simulink model "test_zumo_orientation_ketan"  (R2014b)
settings: Solver=ode3  StartTime=0.0  StopTime=10.0  RelTol=1e-3
InitFcn:
  | prepareCurrentFolderForZumo;
  | load MagnetometerBus;
libraries: arduinolib x2, etargetslib x2, ZumoBotLib x1
settings Model: ExtModeTrigDuration=2  Creator=sandip  LastModifiedBy=sandip
settings OptimizationCC: OptimizeModelRefInitCode=on  LifeSpan=1
settings DebuggingCC: UnderspecifiedInitializationDetection=Classic  MergeDetectMultiDrivingBlocksExec=none  SolverPrmCheckMsg=none
settings HardwareCC: ProdBitPerInt=16  ProdBitPerPointer=8  ProdIntDivRoundTo=Zero  ProdEndianess=LittleEndian  ProdWordSize=8  ProdHWDeviceType=Atmel->AVR
settings RTWCC: SystemTargetFile=realtime.tlc  GenerateMakefile=off  TemplateMakefile=realtime.tmf  Description=Run on Target Hardware  RTWVerbose=off  ProcessScript=realtime_make_rtw_hook
settings STFCustomTargetCC: TargetLibSuffix=.a  GenerateSampleERTMain=on  ERTCustomFileBanners=on  SupportNonInlinedSFcns=off  SupportVariableSizeSignals=on  MATLABClassNameForMDSCustomization=Simulink.SoftwareTarget.ERTCustomization  GRTInterface=off  SystemTargetFile=realtime.tlc
settings ERTTargetCC: GenerateSampleERTMain=on  ParMdlRefBuildCompliant=off  CompOptLevelCompliant=off  ConcurrentExecutionCompliant=off  CombineOutputUpdateFcns=off  ERTFirstTimeCompliant=off  SupportContinuousTime=on  SupportVariableSizeSignals=on  ModelStepFunctionPrototypeControlCompliant=off  CPPClassGenCompliant=off  ExtModeTransport=3  ExtModeMexFile=ext_serial_win32_comm  ExtModeMexArgs=0 1 9600  InlinedParameterPlacement=NonHierarchical  ERTSrcFileBannerTemplate=realtime_code_template.cgt  ERTHdrFileBannerTemplate=realtime_code_template.cgt  ERTDataSrcFileTemplate=realtime_code_template.cgt  ERTDataHdrFileTemplate=realtime_code_template.cgt  ERTCustomFileTemplate=realtime_file_process.tlc

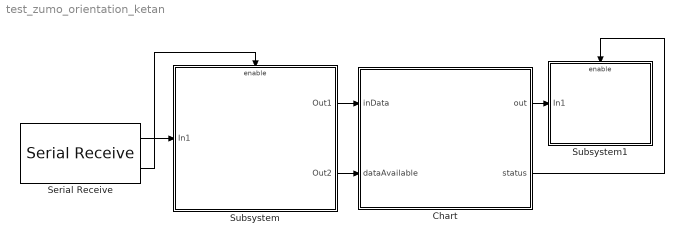
== system test_zumo_orientation_ketan ==
  Chart : Stateflow chart  TreatAsAtomicUnit=on
  Serial Receive : arduinolib/Serial Receive  portNumber=0  showOutStatus=on  sampleTime=0.01  blockPlatform=arduino
  Subsystem : Subsystem
  Subsystem1 : Subsystem
  wires:
  Serial Receive/2 -> Subsystem/Enable
  Subsystem/1(Out1) -> Chart/1(inData)
  Subsystem/2(Out2) -> Chart/2(dataAvailable)
  Chart/1(out) -> Subsystem1/1(In1)
  Chart/2(status) -> Subsystem1/Enable
  Serial Receive/1 -> Subsystem/1(In1)

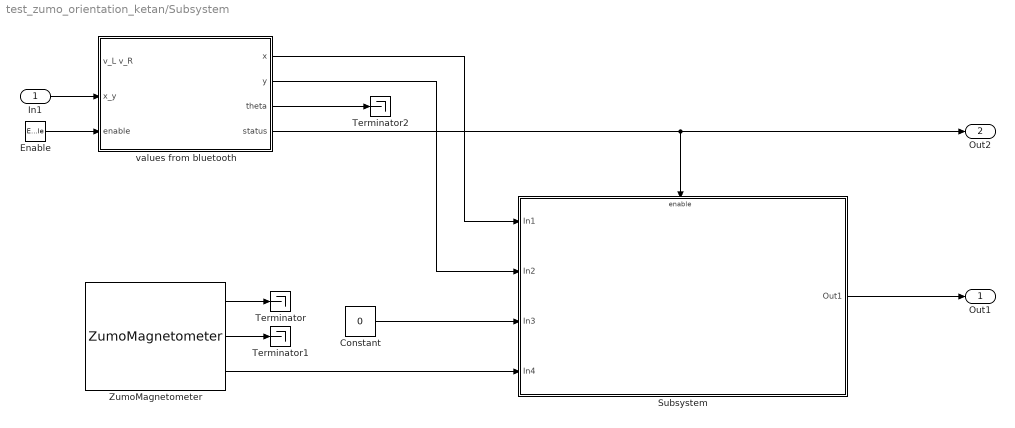
== system test_zumo_orientation_ketan/Subsystem ==
  In1 : Inport
  Enable : EnablePort  ShowOutputPort=on
  Constant : Constant  Value=0
  Subsystem : Subsystem
  Terminator : Terminator
  Terminator1 : Terminator
  Terminator2 : Terminator
  ZumoMagnetometer : ZumoBotLib/ZumoMagnetometer  sampletime_lsm=0.01  debug_lsm=off  minX_lsm=-2048  maxX_lsm=2048  minY_lsm=-2048  maxY_lsm=2048  minZ_lsm=-4096  maxZ_lsm=4096
      link override S-Function Builder: Parameters=sampletime_lsm,boolean(debug_lsm),minX_lsm,maxX_lsm,minY_lsm,maxY_lsm,minZ_lsm,boolean(maxZ_lsm)
  "values from bluetooth " : Subsystem  VariantControl=bluetoothComm==1
  Out1 : Outport
  Out2 : Outport  Port=2  OutputWhenDisabled=reset  InitialOutput=0
  wires:
  ZumoMagnetometer/2 -> Terminator1/1
  ZumoMagnetometer/1 -> Terminator/1
  "values from bluetooth "/3(theta) -> Terminator2/1
  In1/1 -> "values from bluetooth "/2(x_y)
  "values from bluetooth "/1(x) -> Subsystem/1(In1)
  "values from bluetooth "/2(y) -> Subsystem/2(In2)
  Constant/1 -> Subsystem/3(In3)
  ZumoMagnetometer/3 -> Subsystem/4(In4)
  "values from bluetooth "/4(status) -> Subsystem/Enable, Out2/1
  Subsystem/1(Out1) -> Out1/1
  Enable/1 -> "values from bluetooth "/3(enable)

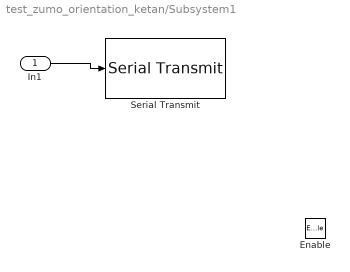
== system test_zumo_orientation_ketan/Subsystem1 ==
  In1 : Inport
  Enable : EnablePort
  Serial Transmit : arduinolib/Serial Transmit  portNumber=0  blockPlatform=arduino
  wires:
  In1/1 -> Serial Transmit/1

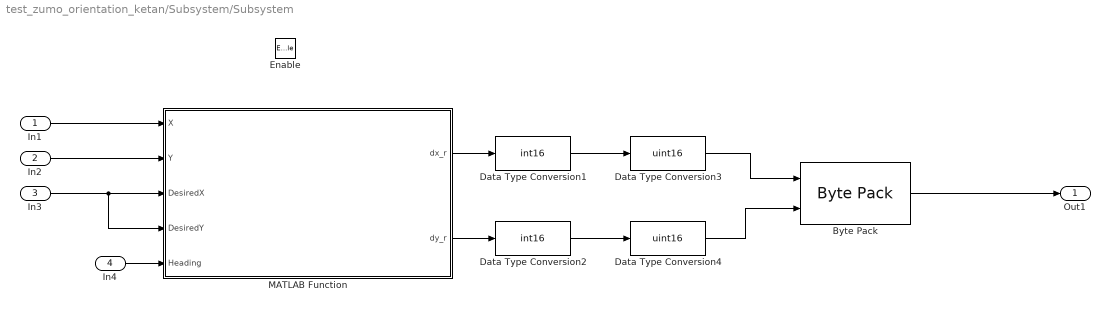
== system test_zumo_orientation_ketan/Subsystem/Subsystem ==
  In1 : Inport
  In2 : Inport  Port=2
  In3 : Inport  Port=3
  In4 : Inport  Port=4
  Enable : EnablePort
  Byte Pack : etargetslib/Byte Pack  datatypes={'uint16','uint16'}  byteAlign=1
  Data Type Conversion1 : DataTypeConversion  OutDataTypeStr=int16
  Data Type Conversion2 : DataTypeConversion  OutDataTypeStr=int16
  Data Type Conversion3 : DataTypeConversion  OutDataTypeStr=uint16  ConvertRealWorld=Stored Integer (SI)
  Data Type Conversion4 : DataTypeConversion  OutDataTypeStr=uint16  ConvertRealWorld=Stored Integer (SI)
  MATLAB Function : MATLAB Function  TreatAsAtomicUnit=on
  Out1 : Outport
  wires:
  In3/1 -> MATLAB Function/4(DesiredY), MATLAB Function/3(DesiredX)
  Data Type Conversion2/1 -> Data Type Conversion4/1
  Data Type Conversion1/1 -> Data Type Conversion3/1
  Byte Pack/1 -> Out1/1
  Data Type Conversion3/1 -> Byte Pack/1
  Data Type Conversion4/1 -> Byte Pack/2
  MATLAB Function/1(dx_r) -> Data Type Conversion1/1
  MATLAB Function/2(dy_r) -> Data Type Conversion2/1
  In2/1 -> MATLAB Function/2(Y)
  In1/1 -> MATLAB Function/1(X)
  In4/1 -> MATLAB Function/5(Heading)

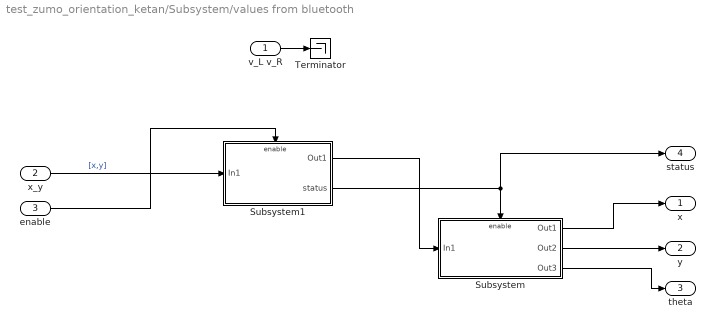
== system test_zumo_orientation_ketan/Subsystem/values from bluetooth  ==
  v_L v_R : Inport
  x_y : Inport  Port=2
  enable : Inport  Port=3
  Subsystem : Subsystem
  Subsystem1 : Subsystem
  Terminator : Terminator
  x : Outport
  y : Outport  Port=2
  theta : Outport  Port=3
  status : Outport  Port=4
  wires:
  v_L v_R/1 -> Terminator/1
  Subsystem/3(Out3) -> theta/1
  x_y/1 -> Subsystem1/1(In1)  "[x,y]"
  Subsystem1/1(Out1) -> Subsystem/1(In1)
  Subsystem/1(Out1) -> x/1
  Subsystem/2(Out2) -> y/1
  Subsystem1/2(status) -> Subsystem/Enable, status/1
  enable/1 -> Subsystem1/Enable

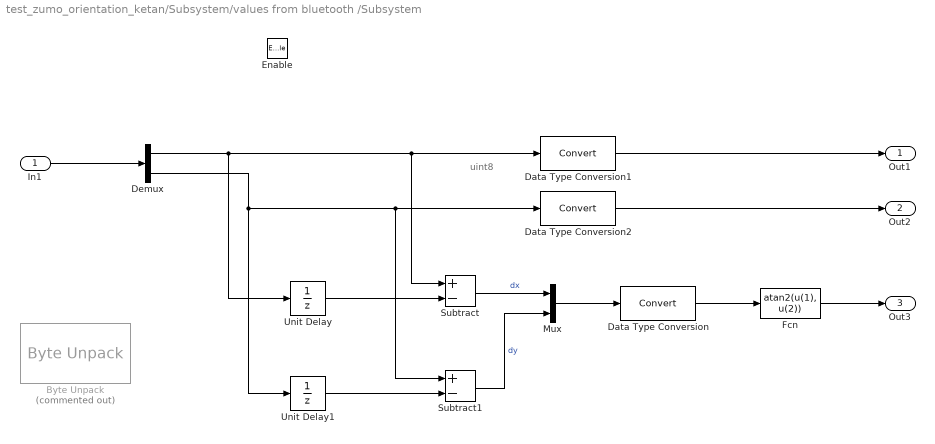
== system test_zumo_orientation_ketan/Subsystem/values from bluetooth /Subsystem ==
  note: uint8
  In1 : Inport
  Enable : EnablePort
  Byte Unpack : etargetslib/Byte Unpack  Commented=on  dimensions={1,1}  datatypes={'uint16', 'uint16'}  byteAlign=1
  Data Type Conversion : DataTypeConversion
  Data Type Conversion1 : DataTypeConversion
  Data Type Conversion2 : DataTypeConversion
  Demux : Demux  Outputs=2
  Fcn : Fcn  Expr=atan2(u(1), u(2))
  Mux : Mux  Inputs=2
  Subtract : Sum  Inputs=+-
  Subtract1 : Sum  Inputs=+-
  Unit Delay : UnitDelay  SampleTime=-1
  Unit Delay1 : UnitDelay  SampleTime=-1
  Out1 : Outport
  Out2 : Outport  Port=2
  Out3 : Outport  Port=3
  wires:
  Demux/1 -> Unit Delay/1, Data Type Conversion1/1, Subtract/1
  Demux/2 -> Unit Delay1/1, Data Type Conversion2/1, Subtract1/1
  Subtract1/1 -> Mux/2  "dy"
  Mux/1 -> Data Type Conversion/1
  Subtract/1 -> Mux/1  "dx"
  Fcn/1 -> Out3/1
  Unit Delay/1 -> Subtract/2
  Unit Delay1/1 -> Subtract1/2
  In1/1 -> Demux/1
  Data Type Conversion/1 -> Fcn/1
  Data Type Conversion1/1 -> Out1/1
  Data Type Conversion2/1 -> Out2/1

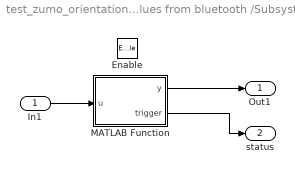
== system test_zumo_orientation_ketan/Subsystem/values from bluetooth /Subsystem1 ==
  In1 : Inport
  Enable : EnablePort
  MATLAB Function : MATLAB Function  TreatAsAtomicUnit=on
  Out1 : Outport
  status : Outport  Port=2
  wires:
  In1/1 -> MATLAB Function/1(u)
  MATLAB Function/1(y) -> Out1/1
  MATLAB Function/2(trigger) -> status/1

== matlab function test_zumo_orientation_ketan/Subsystem/values from bluetooth /Subsystem1/MATLAB Function ==
  data: u input; y output; trigger output
function [y,trigger] = fcn(u)
%#codegen
persistent data count
if isempty(data)
    data = zeros(2,1,'uint8');
    count = 1;
end
trigger = 0;
data(count) = u;
count = count + 1;
if count > 2
    trigger = 1;
    count = 1;
end

y = data;

== stateflow chart test_zumo_orientation_ketan/Chart ==
  state Wait
    entry: status = 0;
  state initBuffer
    entry:
    buffer = inData;
    status = 0;
  state buffer1
    entry: out = buffer(1);
    status = 1;
  state buffer2
    entry: out = buffer(2);
    status = 1;
  state buffer3
    entry: out = buffer(3);
    status = 1;
  state buffer4
    entry: out = buffer(4);
    status = 1;
  (default) -> Wait
  buffer4 -> Wait
  Wait -> initBuffer : [dataAvailable > 0]
  initBuffer -> buffer1
  buffer1 -> buffer2
  buffer2 -> buffer3
  buffer3 -> buffer4
  data: inData input; dataAvailable input; buffer local uint8 size=4; out output uint8; status output

== matlab function test_zumo_orientation_ketan/Subsystem/Subsystem/MATLAB Function ==
  data: X input; dx_r output; Y input; DesiredX input; DesiredY input; Heading input; dy_r output
function [dx_r, dy_r] = moveForward(X,Y,DesiredX,DesiredY,Heading)

persistent R_mc 
%dx_c = DesiredX - X;
%dy_c = DesiredY - Y;
dx_c = X;
dy_c = Y;

heading = Heading * (pi/180);
%R_rm = RotZ(Heading*pi/180);
R_rm = [cos(heading),-sin(heading);sin(heading),cos(heading)];
%R_mr = R_rm';

%R_rc = [1 0;0 -1];

if isempty(R_mc)
    R_mc = [cos(-heading),-sin(-heading);sin(-heading),cos(-heading)] * [1 0;0 -1];
end

d_r = R_rm*R_mc*[dx_c;dy_c];
dx_r = d_r(1);
dy_r = d_r(2);
